simulink model "AFS_VDDrftComp"  (R2016b)
settings: configuration reference "CodeGenConfigSet" (kept outside this file)
values from neighbouring files (symbols this model uses):
  AFS_aOvrnAdjMax_C = Calibration.Parameter    [init_AFS_VDDrftComp.m]    (also in init_AFS_VDDrftComp_SIL.m = Simulink.Parameter)
  AFS_aOvrnAdjMin_C = Calibration.Parameter    [init_AFS_VDDrftComp.m]    (also in init_AFS_VDDrftComp_SIL.m = Simulink.Parameter)
  AFS_dmIdlAirMsLim_C = Calibration.Parameter    [init_AFS_VDDrftComp.m]    (also in init_AFS_VDDrftComp_SIL.m = Simulink.Parameter)
  AFS_dmLdAirMsLim_C = Calibration.Parameter    [init_AFS_VDDrftComp.m]    (also in init_AFS_VDDrftComp_SIL.m = Simulink.Parameter)
  AFS_dnEngLdAdjThresHi_C = Calibration.Parameter    [init_AFS_VDDrftComp.m]    (also in init_AFS_VDDrftComp_SIL.m = Simulink.Parameter)
  AFS_dpLdAdjThresHi_C = Calibration.Parameter    [init_AFS_VDDrftComp.m]    (also in init_AFS_VDDrftComp_SIL.m = Simulink.Parameter)
  AFS_dqLdAdjThresHi_C = Calibration.Parameter    [init_AFS_VDDrftComp.m]    (also in init_AFS_VDDrftComp_SIL.m = Simulink.Parameter)
  AFS_drWtPenDetThresHi_C = Calibration.Parameter    [init_AFS_VDDrftComp.m]    (also in init_AFS_VDDrftComp_SIL.m = Simulink.Parameter)
  AFS_facAdjPlausDiff_C = Calibration.Parameter    [init_AFS_VDDrftComp.m]    (also in init_AFS_VDDrftComp_SIL.m = Simulink.Parameter)
  AFS_facAirMsPT1_C = Calibration.Parameter    [init_AFS_VDDrftComp.m]    (also in init_AFS_VDDrftComp_SIL.m = Simulink.Parameter)
  AFS_facBstPresPT1_C = Calibration.Parameter    [init_AFS_VDDrftComp.m]    (also in init_AFS_VDDrftComp_SIL.m = Simulink.Parameter)
  AFS_facCorExtpIdl_CUR = Calibration.Parameter    [init_AFS_VDDrftComp.m]    (also in init_AFS_VDDrftComp_SIL.m = Simulink.Parameter)
  AFS_facCorExtpIdl_CURX = Calibration.Parameter    [init_AFS_VDDrftComp.m]    (also in init_AFS_VDDrftComp_SIL.m = Simulink.Parameter)
  AFS_facCorExtpLd_CUR = Calibration.Parameter    [init_AFS_VDDrftComp.m]    (also in init_AFS_VDDrftComp_SIL.m = Simulink.Parameter)
  AFS_facCorExtpLd_CURX = Calibration.Parameter    [init_AFS_VDDrftComp.m]    (also in init_AFS_VDDrftComp_SIL.m = Simulink.Parameter)
  AFS_facCorFacPT1_C = Calibration.Parameter    [init_AFS_VDDrftComp.m]    (also in init_AFS_VDDrftComp_SIL.m = Simulink.Parameter)
  AFS_facIdlAdjPlausMax_C = Calibration.Parameter    [init_AFS_VDDrftComp.m]    (also in init_AFS_VDDrftComp_SIL.m = Simulink.Parameter)
  AFS_facIdlAdjValMax_C = Calibration.Parameter    [init_AFS_VDDrftComp.m]    (also in init_AFS_VDDrftComp_SIL.m = Simulink.Parameter)
  AFS_facIdlAdjValMin_C = Calibration.Parameter    [init_AFS_VDDrftComp.m]    (also in init_AFS_VDDrftComp_SIL.m = Simulink.Parameter)
  AFS_facIdlAdjValStepLim_C = Calibration.Parameter    [init_AFS_VDDrftComp.m]    (also in init_AFS_VDDrftComp_SIL.m = Simulink.Parameter)
  AFS_facLdAdjPlausMin_C = Calibration.Parameter    [init_AFS_VDDrftComp.m]    (also in init_AFS_VDDrftComp_SIL.m = Simulink.Parameter)
  AFS_facLdAdjValMax_C = Calibration.Parameter    [init_AFS_VDDrftComp.m]    (also in init_AFS_VDDrftComp_SIL.m = Simulink.Parameter)
  AFS_facLdAdjValMin_C = Calibration.Parameter    [init_AFS_VDDrftComp.m]    (also in init_AFS_VDDrftComp_SIL.m = Simulink.Parameter)
  AFS_facLdAdjValStepLim_C = Calibration.Parameter    [init_AFS_VDDrftComp.m]    (also in init_AFS_VDDrftComp_SIL.m = Simulink.Parameter)
  AFS_facLoThresIdlAdjVal_C = Calibration.Parameter    [init_AFS_VDDrftComp.m]    (also in init_AFS_VDDrftComp_SIL.m = Simulink.Parameter)
  AFS_facLoThresLdAdjVal_C = Calibration.Parameter    [init_AFS_VDDrftComp.m]    (also in init_AFS_VDDrftComp_SIL.m = Simulink.Parameter)
  AFS_facnEngPT1_C = Calibration.Parameter    [init_AFS_VDDrftComp.m]    (also in init_AFS_VDDrftComp_SIL.m = Simulink.Parameter)
  AFS_facQntCurrPT1_C = Calibration.Parameter    [init_AFS_VDDrftComp.m]    (also in init_AFS_VDDrftComp_SIL.m = Simulink.Parameter)
  AFS_facWtPenDetPT1_C = Calibration.Parameter    [init_AFS_VDDrftComp.m]    (also in init_AFS_VDDrftComp_SIL.m = Simulink.Parameter)
  AFS_nAvrgIdlAdjThresHi_C = Calibration.Parameter    [init_AFS_VDDrftComp.m]    (also in init_AFS_VDDrftComp_SIL.m = Simulink.Parameter)
  AFS_nAvrgIdlAdjThresLo_C = Calibration.Parameter    [init_AFS_VDDrftComp.m]    (also in init_AFS_VDDrftComp_SIL.m = Simulink.Parameter)
  AFS_nOvrnAdjMax_C = Calibration.Parameter    [init_AFS_VDDrftComp.m]    (also in init_AFS_VDDrftComp_SIL.m = Simulink.Parameter)
  AFS_nOvrnAdjMin_C = Calibration.Parameter    [init_AFS_VDDrftComp.m]    (also in init_AFS_VDDrftComp_SIL.m = Simulink.Parameter)
  AFS_numAirDrftComp_C = Calibration.Parameter    [init_AFS_VDDrftComp.m]    (also in init_AFS_VDDrftComp_SIL.m = Simulink.Parameter)
  AFS_numEnvTemp_C = Calibration.Parameter    [init_AFS_VDDrftComp.m]    (also in init_AFS_VDDrftComp_SIL.m = Simulink.Parameter)
  AFS_numOvrnAdjGearMin_C = Calibration.Parameter    [init_AFS_VDDrftComp.m]    (also in init_AFS_VDDrftComp_SIL.m = Simulink.Parameter)
  AFS_pBstAtmDiffLim_C = Calibration.Parameter    [init_AFS_VDDrftComp.m]    (also in init_AFS_VDDrftComp_SIL.m = Simulink.Parameter)
  AFS_pBstLdAdjThresHi_C = Calibration.Parameter    [init_AFS_VDDrftComp.m]    (also in init_AFS_VDDrftComp_SIL.m = Simulink.Parameter)
  AFS_pBstLdAdjThresLo_C = Calibration.Parameter    [init_AFS_VDDrftComp.m]    (also in init_AFS_VDDrftComp_SIL.m = Simulink.Parameter)
  AFS_qCurrIdlAdjThresHi_C = Calibration.Parameter    [init_AFS_VDDrftComp.m]    (also in init_AFS_VDDrftComp_SIL.m = Simulink.Parameter)
  AFS_qCurrIdlAdjThresLo_C = Calibration.Parameter    [init_AFS_VDDrftComp.m]    (also in init_AFS_VDDrftComp_SIL.m = Simulink.Parameter)
  AFS_qWinLdAdjThresHi_CUR = Calibration.Parameter    [init_AFS_VDDrftComp.m]    (also in init_AFS_VDDrftComp_SIL.m = Simulink.Parameter)
  AFS_qWinLdAdjThresHi_CURX = Calibration.Parameter    [init_AFS_VDDrftComp.m]    (also in init_AFS_VDDrftComp_SIL.m = Simulink.Parameter)
  AFS_qWinLdAdjThresLo_CUR = Calibration.Parameter    [init_AFS_VDDrftComp.m]    (also in init_AFS_VDDrftComp_SIL.m = Simulink.Parameter)
  AFS_qWinLdAdjThresLo_CURX = Calibration.Parameter    [init_AFS_VDDrftComp.m]    (also in init_AFS_VDDrftComp_SIL.m = Simulink.Parameter)
  AFS_swtAdjPlausLim_C = Calibration.Parameter    [init_AFS_VDDrftComp.m]    (also in init_AFS_VDDrftComp_SIL.m = Simulink.Parameter)
  AFS_swtAirMsCorRls_C = Calibration.Parameter    [init_AFS_VDDrftComp.m]    (also in init_AFS_VDDrftComp_SIL.m = Simulink.Parameter)
  AFS_swtLdAdjSel_C = Calibration.Parameter    [init_AFS_VDDrftComp.m]    (also in init_AFS_VDDrftComp_SIL.m = Simulink.Parameter)
  AFS_tAirAdjRlsThresHi_C = Calibration.Parameter    [init_AFS_VDDrftComp.m]    (also in init_AFS_VDDrftComp_SIL.m = Simulink.Parameter)
  AFS_tAirAdjRlsThresLo_C = Calibration.Parameter    [init_AFS_VDDrftComp.m]    (also in init_AFS_VDDrftComp_SIL.m = Simulink.Parameter)
  AFS_tEnvAdjRlsThresHi_C = Calibration.Parameter    [init_AFS_VDDrftComp.m]    (also in init_AFS_VDDrftComp_SIL.m = Simulink.Parameter)
  AFS_tEnvAdjRlsThresLo_C = Calibration.Parameter    [init_AFS_VDDrftComp.m]    (also in init_AFS_VDDrftComp_SIL.m = Simulink.Parameter)
  AFS_tiAdjRlsDel_C = Calibration.Parameter    [init_AFS_VDDrftComp.m]    (also in init_AFS_VDDrftComp_SIL.m = Simulink.Parameter)
  AFS_tiIdlAdjRlsDeb = Calibration.Parameter    [init_AFS_VDDrftComp.m]    (also in init_AFS_VDDrftComp_SIL.m = Simulink.Parameter)
  AFS_tiLdAdjRlsDeb = Calibration.Parameter    [init_AFS_VDDrftComp.m]    (also in init_AFS_VDDrftComp_SIL.m = Simulink.Parameter)
  AFS_tiStrtDelAdjRls_C = Calibration.Parameter    [init_AFS_VDDrftComp.m]    (also in init_AFS_VDDrftComp_SIL.m = Simulink.Parameter)
  AFS_tiWtPenDeb = Calibration.Parameter    [init_AFS_VDDrftComp.m]    (also in init_AFS_VDDrftComp_SIL.m = Simulink.Parameter)
  AFS_vOvrnAdjMin_C = Calibration.Parameter    [init_AFS_VDDrftComp.m]    (also in init_AFS_VDDrftComp_SIL.m = Simulink.Parameter)
  AFS_vVehLdAdjThresHi_C = Calibration.Parameter    [init_AFS_VDDrftComp.m]    (also in init_AFS_VDDrftComp_SIL.m = Simulink.Parameter)
  AFS_vVehLdAdjThresLo_C = Calibration.Parameter    [init_AFS_VDDrftComp.m]    (also in init_AFS_VDDrftComp_SIL.m = Simulink.Parameter)
  AIRCTL_DRFTCOMP = fi(5,State_uint8)    [init_AFS_VDDrftComp.m]    (also in init_AFS_VDDrftComp_SIL.m)
undefined symbols (not defined in the file or in its folder): AFS_VDDrftComp_DT, Switch_conv
libraries: simulink x82, CXLib x13
(part 2 of 2)

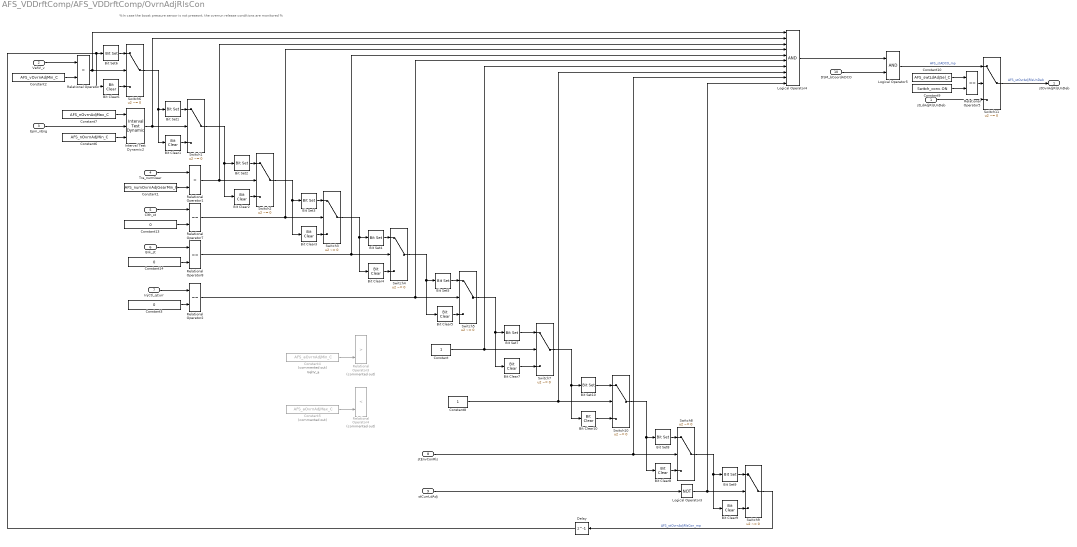
== system AFS_VDDrftComp/AFS_VDDrftComp/OvrnAdjRlsCon ==
  note: VehV_a
  note: %In case the boost pressure sensor is not presesnt, the overrun release conditions are monitored %
  stLdAdjRlsUnDeb : Inport
  VehV_v : Inport  Port=2
  Epm_nEng : Inport  Port=3
  Tra_numGear : Inport  Port=4
  Clth_st : Inport  Port=5
  Brk_st : Inport  Port=6
  InjCtl_qCurr : Inport  Port=7
  stEnvConRls : Inport  Port=8
  stCurrLdAdj : Inport  Port=9
  DSM_bCoordADCO : Inport  Port=10
  Bit Clear1 : simulink/Logic and Bit Operations/Bit Clear  iBit=1
  Bit Clear10 : simulink/Logic and Bit Operations/Bit Clear  iBit=7
  Bit Clear2 : simulink/Logic and Bit Operations/Bit Clear  iBit=2
  Bit Clear3 : simulink/Logic and Bit Operations/Bit Clear  iBit=3
  Bit Clear4 : simulink/Logic and Bit Operations/Bit Clear  iBit=4
  Bit Clear5 : simulink/Logic and Bit Operations/Bit Clear  iBit=5
  Bit Clear6 : simulink/Logic and Bit Operations/Bit Clear  iBit=0
  Bit Clear7 : simulink/Logic and Bit Operations/Bit Clear  iBit=6
  Bit Clear8 : simulink/Logic and Bit Operations/Bit Clear  iBit=8
  Bit Clear9 : simulink/Logic and Bit Operations/Bit Clear  iBit=9
  Bit Set1 : simulink/Logic and Bit Operations/Bit Set  iBit=1
  Bit Set10 : simulink/Logic and Bit Operations/Bit Set  iBit=7
  Bit Set2 : simulink/Logic and Bit Operations/Bit Set  iBit=2
  Bit Set3 : simulink/Logic and Bit Operations/Bit Set  iBit=3
  Bit Set4 : simulink/Logic and Bit Operations/Bit Set  iBit=4
  Bit Set5 : simulink/Logic and Bit Operations/Bit Set  iBit=5
  Bit Set6 : simulink/Logic and Bit Operations/Bit Set  iBit=0
  Bit Set7 : simulink/Logic and Bit Operations/Bit Set  iBit=6
  Bit Set8 : simulink/Logic and Bit Operations/Bit Set  iBit=8
  Bit Set9 : simulink/Logic and Bit Operations/Bit Set  iBit=9
  Constant : Constant  OutDataTypeStr=boolean
  Constant1 : Constant  Value=AFS_numOvrnAdjGearMin_C
  Constant10 : Constant  Value=AFS_swtLdAdjSel_C
  Constant13 : Constant  Value=0  OutDataTypeStr=Inherit: Inherit via back propagation
  Constant14 : Constant  Value=0  OutDataTypeStr=Inherit: Inherit via back propagation
  Constant2 : Constant  Value=AFS_vOvrnAdjMin_C
  Constant3 : Constant  Value=0  OutDataTypeStr=Inherit: Inherit via back propagation
  Constant4 : Constant  Commented=on  Value=AFS_aOvrnAdjMin_C
  Constant5 : Constant  Commented=on  Value=AFS_aOvrnAdjMax_C
  Constant6 : Constant  Value=AFS_nOvrnAdjMin_C
  Constant7 : Constant  Value=AFS_nOvrnAdjMax_C
  Constant8 : Constant  OutDataTypeStr=boolean
  Constant9 : Constant  Value=Switch_conv.ON
  Delay : Delay  DelayLength=1  InitialCondition=0
  Interval Test Dynamic2 : simulink/Logic and Bit Operations/Interval Test Dynamic  IntervalClosedRight=off  IntervalClosedLeft=off  OutDataTypeStr=boolean
  Logical Operator3 : Logic  Operator=NOT  Inputs=5  AllPortsSameDT=off  OutDataTypeStr=boolean
  Logical Operator4 : Logic  Inputs=10  AllPortsSameDT=off  OutDataTypeStr=boolean
  Logical Operator5 : Logic  AllPortsSameDT=off  OutDataTypeStr=boolean
  Relational Operator : RelationalOperator  Operator=>  OutDataTypeStr=boolean  RndMeth=Simplest
  Relational Operator1 : RelationalOperator  Operator=>  OutDataTypeStr=boolean  RndMeth=Simplest
  Relational Operator2 : RelationalOperator  Operator===  OutDataTypeStr=boolean  RndMeth=Simplest  InputSameDT=on
  Relational Operator3 : RelationalOperator  Commented=on  Operator=>  OutDataTypeStr=boolean  RndMeth=Simplest  InputSameDT=on
  Relational Operator4 : RelationalOperator  Commented=on  Operator=<  OutDataTypeStr=boolean  RndMeth=Simplest  InputSameDT=on
  Relational Operator5 : RelationalOperator  Operator===  OutDataTypeStr=boolean  RndMeth=Simplest
  Relational Operator7 : RelationalOperator  Operator===  OutDataTypeStr=boolean  RndMeth=Simplest  InputSameDT=on
  Relational Operator8 : RelationalOperator  Operator===  OutDataTypeStr=boolean  RndMeth=Simplest  InputSameDT=on
  Switch{1..11} (11 alike) : Switch  Criteria=u2 ~= 0  OutDataTypeStr=Inherit: Inherit via back propagation  SaturateOnIntegerOverflow=on
  stOvrAdjRlsUnDeb : Outport
  wires:
  Constant14/1 -> Relational Operator8/2
  Brk_st/1 -> Relational Operator8/1
  Constant13/1 -> Relational Operator7/2
  Switch11/1 -> stOvrAdjRlsUnDeb/1  "AFS_stOvrAdjRlsUnDeb"
  Constant10/1 -> Relational Operator5/1
  Relational Operator5/1 -> Switch11/2
  Constant9/1 -> Relational Operator5/2
  stLdAdjRlsUnDeb/1 -> Switch11/3
  Logical Operator5/1 -> Switch11/1  "AFS_stADCO_mp"
  Logical Operator4/1 -> Logical Operator5/1
  Delay/1 -> Bit Set6/1, Bit Clear6/1
  Switch9/1 -> Delay/1  "AFS_stOvrnAdjRlsCon_mp"
  Switch10/1 -> Bit Set8/1, Bit Clear8/1
  Constant5/1 -> Relational Operator4/2
  Switch7/1 -> Bit Clear10/1, Bit Set10/1
  Bit Set10/1 -> Switch10/1
  Bit Clear10/1 -> Switch10/3
  Switch8/1 -> Bit Clear9/1, Bit Set9/1
  Logical Operator3/1 -> Switch9/2, Logical Operator4/10
  Bit Set9/1 -> Switch9/1
  Bit Clear9/1 -> Switch9/3
  stCurrLdAdj/1 -> Logical Operator3/1
  stEnvConRls/1 -> Switch8/2, Logical Operator4/9
  Bit Set8/1 -> Switch8/1
  Bit Clear8/1 -> Switch8/3
  Switch5/1 -> Bit Set7/1, Bit Clear7/1
  Bit Set7/1 -> Switch7/1
  Bit Clear7/1 -> Switch7/3
  Constant4/1 -> Relational Operator3/2
  Switch4/1 -> Bit Clear5/1, Bit Set5/1
  Relational Operator2/1 -> Switch5/2, Logical Operator4/6
  Bit Set5/1 -> Switch5/1
  Bit Clear5/1 -> Switch5/3
  InjCtl_qCurr/1 -> Relational Operator2/1
  Constant3/1 -> Relational Operator2/2
  Switch3/1 -> Bit Set4/1, Bit Clear4/1
  Relational Operator8/1 -> Switch4/2, Logical Operator4/5
  Bit Set4/1 -> Switch4/1
  Bit Clear4/1 -> Switch4/3
  Switch2/1 -> Bit Clear3/1, Bit Set3/1
  Relational Operator7/1 -> Switch3/2, Logical Operator4/4
  Bit Set3/1 -> Switch3/1
  Bit Clear3/1 -> Switch3/3
  Clth_st/1 -> Relational Operator7/1
  Switch1/1 -> Bit Set2/1, Bit Clear2/1
  Relational Operator1/1 -> Switch2/2, Logical Operator4/3
  Bit Set2/1 -> Switch2/1
  Bit Clear2/1 -> Switch2/3
  Tra_numGear/1 -> Relational Operator1/1
  Constant1/1 -> Relational Operator1/2
  Switch6/1 -> Bit Set1/1, Bit Clear1/1
  Interval Test Dynamic2/1 -> Switch1/2, Logical Operator4/2
  Bit Set1/1 -> Switch1/1
  Bit Clear1/1 -> Switch1/3
  Epm_nEng/1 -> Interval Test Dynamic2/2
  Constant6/1 -> Interval Test Dynamic2/3
  Constant7/1 -> Interval Test Dynamic2/1
  Relational Operator/1 -> Switch6/2, Logical Operator4/1
  Bit Set6/1 -> Switch6/1
  Bit Clear6/1 -> Switch6/3
  VehV_v/1 -> Relational Operator/1
  Constant2/1 -> Relational Operator/2
  DSM_bCoordADCO/1 -> Logical Operator5/2
  Constant/1 -> Logical Operator4/7, Switch7/2
  Constant8/1 -> Logical Operator4/8, Switch10/2

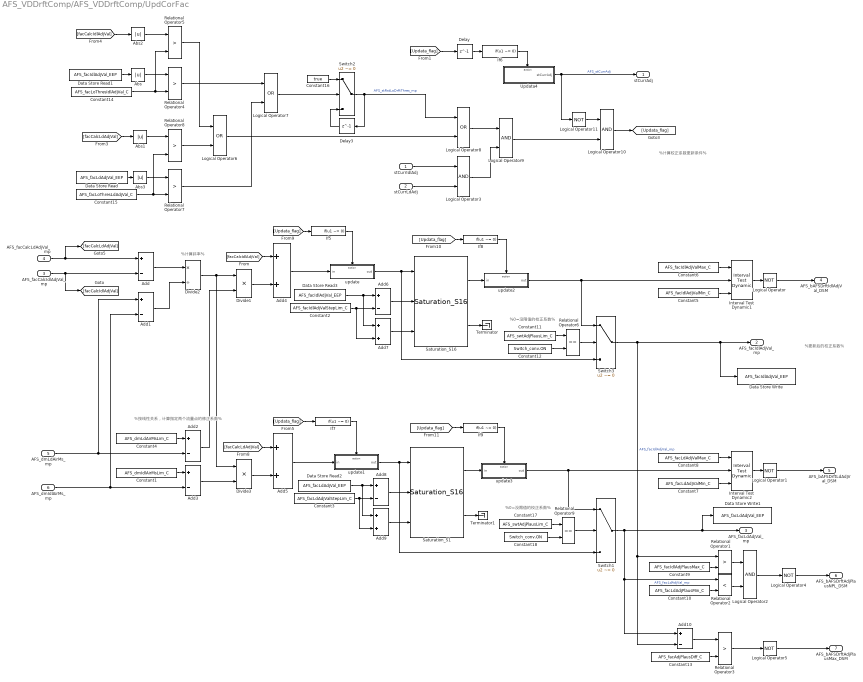
== system AFS_VDDrftComp/AFS_VDDrftComp/UpdCorFac ==
  note: %0=没限值的校正系数%
  note: %计算斜率%
  note: %0=没限值的校正系数%
  note: %计算校正系数更新条件%
  note: %更新后的校正系数%
  note: %按线性关系，计算指定两个流量点的修正系数%
  stCurrIdlAdj : Inport
  stCurrLdAdj : Inport  Port=2
  AFS_facCalcIdlAdjVal_mp : Inport  Port=3
  AFS_facCalcLdAdjVal_mp : Inport  Port=4
  AFS_dmLdAirMs_mp : Inport  Port=5
  AFS_dmIdlAirMs_mp : Inport  Port=6
  Abs{,1..3} (4 alike) : Abs  SaturateOnIntegerOverflow=on
  Add{,2..3,6,8,10} (6 alike) : Sum  Inputs=+-  OutDataTypeStr=Inherit: Inherit via back propagation  SaturateOnIntegerOverflow=on  InputSameDT=on
  Add1 : Sum  Inputs=+-  SaturateOnIntegerOverflow=on  InputSameDT=on
  Add{4..5,7,9} (4 alike) : Sum  OutDataTypeStr=Inherit: Inherit via back propagation  SaturateOnIntegerOverflow=on  InputSameDT=on
  Constant1 : Constant  Value=AFS_dmIdlAirMsLim_C
  Constant10 : Constant  Value=AFS_facLdAdjPlausMin_C
  Constant11 : Constant  Value=AFS_swtAdjPlausLim_C
  Constant12 : Constant  Value=Switch_conv.ON
  Constant13 : Constant  Value=AFS_facAdjPlausDiff_C
  Constant14 : Constant  Value=AFS_facLoThresIdlAdjVal_C
  Constant15 : Constant  Value=AFS_facLoThresLdAdjVal_C
  Constant16 : Constant  Value=true  OutDataTypeStr=Inherit: Inherit via back propagation
  Constant17 : Constant  Value=AFS_swtAdjPlausLim_C
  Constant18 : Constant  Value=Switch_conv.ON
  Constant2 : Constant  Value=AFS_facIdlAdjValStepLim_C
  Constant3 : Constant  Value=AFS_facLdAdjValStepLim_C
  Constant4 : Constant  Value=AFS_dmLdAirMsLim_C
  Constant5 : Constant  Value=AFS_facIdlAdjValMin_C
  Constant6 : Constant  Value=AFS_facIdlAdjValMax_C
  Constant7 : Constant  Value=AFS_facLdAdjValMin_C
  Constant8 : Constant  Value=AFS_facLdAdjValMax_C
  Constant9 : Constant  Value=AFS_facIdlAdjPlausMax_C
  Data Store Read : DataStoreRead  DataStoreName=AFS_facLdAdjVal_EEP
  Data Store Read1 : DataStoreRead  DataStoreName=AFS_facIdlAdjVal_EEP
  Data Store Read2 : DataStoreRead  DataStoreName=AFS_facLdAdjVal_EEP
  Data Store Read3 : DataStoreRead  DataStoreName=AFS_facIdlAdjVal_EEP
  Data Store Write : DataStoreWrite  DataStoreName=AFS_facIdlAdjVal_EEP
  Data Store Write1 : DataStoreWrite  DataStoreName=AFS_facLdAdjVal_EEP
  Delay : Delay  DelayLength=1  InitialCondition=0
  Delay3 : Delay  DelayLength=1  InitialCondition=0
  Divide1 : Product  Inputs=**  OutDataTypeStr=Inherit: Inherit via back propagation  SaturateOnIntegerOverflow=on
  Divide2 : Product  Inputs=*/  SaturateOnIntegerOverflow=on
  Divide3 : Product  Inputs=**  OutDataTypeStr=Inherit: Inherit via back propagation  SaturateOnIntegerOverflow=on
  If{5..9} (5 alike) : If  IfExpression=u1 ~= 0  ShowElse=off
  Interval Test Dynamic1 : simulink/Logic and Bit Operations/Interval Test Dynamic  IntervalClosedRight=on  IntervalClosedLeft=on  OutDataTypeStr=boolean
  Interval Test Dynamic2 : simulink/Logic and Bit Operations/Interval Test Dynamic  IntervalClosedRight=on  IntervalClosedLeft=on  OutDataTypeStr=boolean
  Logical Operator{,1,4..5,11} (5 alike) : Logic  Operator=NOT  AllPortsSameDT=off  OutDataTypeStr=boolean
  Logical Operator{2..3,9..10} (4 alike) : Logic  OutDataTypeStr=boolean
  Logical Operator6 : Logic  Operator=OR  OutDataTypeStr=boolean
  Logical Operator7 : Logic  Operator=OR  OutDataTypeStr=boolean
  Logical Operator8 : Logic  Operator=OR  OutDataTypeStr=boolean
  Relational Operator{1,3..5,7..8} (6 alike) : RelationalOperator  Operator=>  OutDataTypeStr=boolean  RndMeth=Simplest  InputSameDT=on
  Relational Operator2 : RelationalOperator  Operator=<  OutDataTypeStr=boolean  RndMeth=Simplest  InputSameDT=on
  Relational Operator6 : RelationalOperator  Operator===  OutDataTypeStr=boolean  RndMeth=Simplest  InputSameDT=on
  Relational Operator9 : RelationalOperator  Operator===  OutDataTypeStr=boolean  RndMeth=Simplest  InputSameDT=on
  Saturation_S1 : CXLib/Saturation_S16
  Saturation_S16 : CXLib/Saturation_S16
  Switch1 : Switch  Criteria=u2 ~= 0  OutDataTypeStr=Inherit: Inherit via back propagation  SaturateOnIntegerOverflow=on  InputSameDT=on
  Switch2 : Switch  Criteria=u2 ~= 0  OutDataTypeStr=Inherit: Inherit via back propagation  SaturateOnIntegerOverflow=on  InputSameDT=on
  Switch3 : Switch  Criteria=u2 ~= 0  OutDataTypeStr=Inherit: Inherit via back propagation  SaturateOnIntegerOverflow=on  InputSameDT=on
  Terminator : Terminator
  Terminator1 : Terminator
  Updata4 : Subsystem  TreatAsAtomicUnit=on
  update : Subsystem  TreatAsAtomicUnit=on
  update1 : Subsystem  TreatAsAtomicUnit=on
  update2 : Subsystem  TreatAsAtomicUnit=on
  update3 : Subsystem  TreatAsAtomicUnit=on
  stCurrAdj : Outport
  AFS_facIdlAdjVal_mp : Outport  Port=2
  AFS_facLdAdjVal_mp : Outport  Port=3
  AFS_bAFSDrftIdlAdjVal_DSM : Outport  Port=4
  AFS_bAFSDrftLdAdjVal_DSM : Outport  Port=5
  AFS_bAFSDrftAdjPlausNPL_DSM : Outport  Port=6
  AFS_bAFSDrftAdjPlausMax_DSM : Outport  Port=7
  wires:
  Delay/1 -> If6/1
  Logical Operator11/1 -> Logical Operator10/1
  [Updata_flag] -> Delay/1
  Relational Operator9/1 -> Switch1/2
  Constant17/1 -> Relational Operator9/1
  Constant18/1 -> Relational Operator9/2
  Saturation_S1/1 -> update3/1(in)
  If9/1 -> update3/Action
  Saturation_S16/1 -> update2/1(in)
  If8/1 -> update2/Action
  [Updata_flag] -> If9/1
  [Updata_flag] -> If8/1
  Add9/1 -> Saturation_S1/3
  Add8/1 -> Saturation_S1/2
  update1/1(out) -> Saturation_S1/1, Switch1/3
  Add5/1 -> update1/1(in)
  [Updata_flag] -> If7/1
  If7/1 -> update1/Action
  [facCalcIdlAdjVal] -> Add4/1
  [facCalcLdAdjVal] -> Add5/1
  [Updata_flag] -> If5/1
  If5/1 -> update/Action
  Delay3/1 -> Switch2/3
  Constant16/1 -> Switch2/1
  [facCalcIdlAdjVal] -> Abs2/1
  [facCalcLdAdjVal] -> Abs1/1
  Updata4/1(stCurrAdj) -> stCurrAdj/1, Logical Operator11/1  "AFS_stCurrAdj"
  If6/1 -> Updata4/Action
  Logical Operator10/1 -> [Updata_flag]
  Logical Operator9/1 -> Logical Operator10/2
  Logical Operator3/1 -> Logical Operator9/2
  Logical Operator8/1 -> Logical Operator9/1
  Logical Operator6/1 -> Logical Operator8/2
  Switch2/1 -> Logical Operator8/1, Delay3/1  "AFS_stRstLoDrftThres_mp"
  Logical Operator7/1 -> Switch2/2
  Relational Operator7/1 -> Logical Operator7/2
  Relational Operator4/1 -> Logical Operator7/1
  Relational Operator5/1 -> Logical Operator6/1
  Relational Operator8/1 -> Logical Operator6/2
  Abs3/1 -> Relational Operator7/1
  Abs2/1 -> Relational Operator5/1
  Abs1/1 -> Relational Operator8/1
  Data Store Read/1 -> Abs3/1
  Constant15/1 -> Relational Operator7/2, Relational Operator8/2
  Constant14/1 -> Relational Operator4/2, Relational Operator5/2
  Abs/1 -> Relational Operator4/1
  Data Store Read1/1 -> Abs/1
  Logical Operator5/1 -> AFS_bAFSDrftAdjPlausMax_DSM/1
  Relational Operator3/1 -> Logical Operator5/1
  Constant13/1 -> Relational Operator3/2
  Add10/1 -> Relational Operator3/1
  Logical Operator2/1 -> Logical Operator4/1
  Relational Operator2/1 -> Logical Operator2/2
  Relational Operator1/1 -> Logical Operator2/1
  Constant10/1 -> Relational Operator2/2
  Switch1/1 -> Relational Operator2/1, Add10/1, Data Store Write1/1, AFS_facLdAdjVal_mp/1  "AFS_facLdAdjVal_mp"
  Constant9/1 -> Relational Operator1/2
  Switch3/1 -> Relational Operator1/1, Add10/2, Data Store Write/1, AFS_facIdlAdjVal_mp/1  "AFS_facIdlAdjVal_mp"
  Interval Test Dynamic2/1 -> Logical Operator1/1
  Constant7/1 -> Interval Test Dynamic2/3
  Constant8/1 -> Interval Test Dynamic2/1
  Logical Operator/1 -> AFS_bAFSDrftIdlAdjVal_DSM/1
  Interval Test Dynamic1/1 -> Logical Operator/1
  Constant5/1 -> Interval Test Dynamic1/3
  Constant6/1 -> Interval Test Dynamic1/1
  update/1(out) -> Saturation_S16/1, Switch3/3
  update3/1(out) -> Interval Test Dynamic2/2, Switch1/1
  update2/1(out) -> Switch3/1, Interval Test Dynamic1/2
  Relational Operator6/1 -> Switch3/2
  Constant11/1 -> Relational Operator6/1
  Constant12/1 -> Relational Operator6/2
  Saturation_S1/2 -> Terminator1/1
  Saturation_S16/2 -> Terminator/1
  Constant3/1 -> Add8/2, Add9/2
  Data Store Read2/1 -> Add8/1, Add9/1
  Add7/1 -> Saturation_S16/3
  Add6/1 -> Saturation_S16/2
  Constant2/1 -> Add7/2, Add6/2
  Data Store Read3/1 -> Add6/1, Add7/1
  Add4/1 -> update/1(in)
  Divide3/1 -> Add5/2
  Add3/1 -> Divide3/2
  Divide1/1 -> Add4/2
  Add2/1 -> Divide1/2
  Divide2/1 -> Divide3/1, Divide1/1
  Constant1/1 -> Add3/1
  Constant4/1 -> Add2/1
  Add1/1 -> Divide2/2
  Add/1 -> Divide2/1
  AFS_dmIdlAirMs_mp/1 -> Add3/2, Add1/2
  AFS_dmLdAirMs_mp/1 -> Add1/1, Add2/2
  AFS_facCalcIdlAdjVal_mp/1 -> [facCalcIdlAdjVal], Add/2
  AFS_facCalcLdAdjVal_mp/1 -> Add/1, [facCalcLdAdjVal]
  stCurrLdAdj/1 -> Logical Operator3/2
  stCurrIdlAdj/1 -> Logical Operator3/1
  Logical Operator1/1 -> AFS_bAFSDrftLdAdjVal_DSM/1
  Logical Operator4/1 -> AFS_bAFSDrftAdjPlausNPL_DSM/1

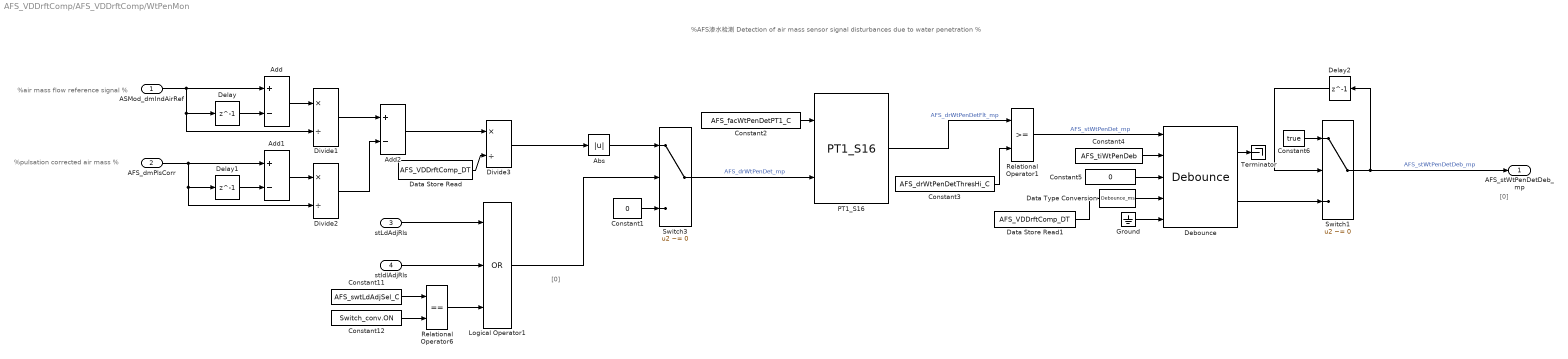
== system AFS_VDDrftComp/AFS_VDDrftComp/WtPenMon ==
  note: %AFS渗水检测
      | Detection of air mass sensor signal disturbances due to water penetration %
  note: %pulsation corrected air mass %
  note: %air mass flow reference signal %
  note: [0]
  note: [0]
  ASMod_dmIndAirRef : Inport
  AFS_dmPlsCorr : Inport  Port=2
  stLdAdjRls : Inport  Port=3
  stIdlAdjRls : Inport  Port=4
  Abs : Abs  SaturateOnIntegerOverflow=on
  Add : Sum  Inputs=+-  OutDataTypeStr=Inherit: Inherit via back propagation  SaturateOnIntegerOverflow=on  InputSameDT=on
  Add1 : Sum  Inputs=+-  OutDataTypeStr=Inherit: Inherit via back propagation  SaturateOnIntegerOverflow=on  InputSameDT=on
  Add2 : Sum  Inputs=+-  SaturateOnIntegerOverflow=on  InputSameDT=on
  Constant1 : Constant  Value=0  OutDataTypeStr=Rmp_1_s
  Constant11 : Constant  Value=AFS_swtLdAdjSel_C
  Constant12 : Constant  Value=Switch_conv.ON
  Constant2 : Constant  Value=AFS_facWtPenDetPT1_C
  Constant3 : Constant  Value=AFS_drWtPenDetThresHi_C
  Constant4 : Constant  Value=AFS_tiWtPenDeb
  Constant5 : Constant  Value=0  OutDataTypeStr=Debounce_ms
  Constant6 : Constant  Value=true  OutDataTypeStr=Inherit: Inherit via back propagation
  Data Store Read : DataStoreRead  DataStoreName=AFS_VDDrftComp_DT
  Data Store Read1 : DataStoreRead  DataStoreName=AFS_VDDrftComp_DT
  Data Type Conversion : DataTypeConversion  OutDataTypeStr=Debounce_ms
  Debounce : CXLib/Debounce
  Delay : Delay  DelayLength=1  InitialCondition=0
  Delay1 : Delay  DelayLength=1  InitialCondition=0
  Delay2 : Delay  DelayLength=1  InitialCondition=0
  Divide1 : Product  Inputs=*/  OutDataTypeStr=Factor  SaturateOnIntegerOverflow=on
  Divide2 : Product  Inputs=*/  OutDataTypeStr=Factor  SaturateOnIntegerOverflow=on
  Divide3 : Product  Inputs=*/  OutDataTypeStr=Inherit: Inherit via back propagation  SaturateOnIntegerOverflow=on
  Ground : Ground
  Logical Operator1 : Logic  Operator=OR  Inputs=3  OutDataTypeStr=boolean
  PT1_S16 : CXLib/PT1_S16
  Relational Operator1 : RelationalOperator  OutDataTypeStr=boolean  RndMeth=Simplest  InputSameDT=on
  Relational Operator6 : RelationalOperator  Operator===  OutDataTypeStr=boolean  RndMeth=Simplest
  Switch1 : Switch  Criteria=u2 ~= 0  OutDataTypeStr=Inherit: Inherit via back propagation  SaturateOnIntegerOverflow=on  InputSameDT=on
  Switch3 : Switch  Criteria=u2 ~= 0  OutDataTypeStr=Inherit: Inherit via back propagation  SaturateOnIntegerOverflow=on  InputSameDT=on
  Terminator : Terminator
  AFS_stWtPenDetDeb_mp : Outport
  wires:
  Debounce/1 -> Terminator/1
  Delay2/1 -> Switch1/2
  Switch1/1 -> Delay2/1, AFS_stWtPenDetDeb_mp/1  "AFS_stWtPenDetDeb_mp"
  Constant6/1 -> Switch1/1
  Debounce/2 -> Switch1/3
  Constant5/1 -> Debounce/3
  Constant4/1 -> Debounce/2
  Data Store Read1/1 -> Data Type Conversion/1
  Ground/1 -> Debounce/5
  Relational Operator1/1 -> Debounce/1  "AFS_stWtPenDet_mp"
  Constant2/1 -> PT1_S16/1
  Switch3/1 -> PT1_S16/2  "AFS_drWtPenDet_mp"
  Constant1/1 -> Switch3/3
  Logical Operator1/1 -> Switch3/2
  Relational Operator6/1 -> Logical Operator1/3
  Constant11/1 -> Relational Operator6/1
  Constant12/1 -> Relational Operator6/2
  Abs/1 -> Switch3/1
  Divide3/1 -> Abs/1
  Data Store Read/1 -> Divide3/2
  Add2/1 -> Divide3/1
  Divide2/1 -> Add2/2
  Add1/1 -> Divide2/1
  AFS_dmPlsCorr/1 -> Add1/1, Delay1/1, Divide2/2
  Delay1/1 -> Add1/2
  Divide1/1 -> Add2/1
  ASMod_dmIndAirRef/1 -> Add/1, Delay/1, Divide1/2
  Add/1 -> Divide1/1
  Delay/1 -> Add/2
  stIdlAdjRls/1 -> Logical Operator1/2
  stLdAdjRls/1 -> Logical Operator1/1
  PT1_S16/1 -> Relational Operator1/1  "AFS_drWtPenDetFlt_mp"
  Constant3/1 -> Relational Operator1/2
  Data Type Conversion/1 -> Debounce/4

== system AFS_VDDrftComp/AFS_VDDrftComp/ AdjRlsEnvCon/AFS_tAirDrftComp_mp ==
  TempSwt : Inport
  Air_tAFS_mp : Inport  Tag=deg  Description=Induction air temperature at the HFM  Port=2
  EnvT_t : Inport  Tag=deg  Description=Environmental temperature  Port=3
  Air_tIntkVUs : Inport  Tag=deg  Description=Intake air temperature upstream of the inlet valve  Port=4
  Data Type Conversion : DataTypeConversion  OutDataTypeStr=uint8
  Multiport Switch : MultiPortSwitch  DataPortOrder=Zero-based contiguous
  AFS_tAirDrftComp_mp : Outport  Tag=deg  Description=Engine temperature field
  wires:
  Multiport Switch/1 -> AFS_tAirDrftComp_mp/1
  Data Type Conversion/1 -> Multiport Switch/1
  TempSwt/1 -> Data Type Conversion/1
  Air_tIntkVUs/1 -> Multiport Switch/4
  Air_tAFS_mp/1 -> Multiport Switch/2
  EnvT_t/1 -> Multiport Switch/3

== system AFS_VDDrftComp/AFS_VDDrftComp/ AdjRlsEnvCon/AFS_tEnvTemp_mp ==
  TempSwt : Inport
  Air_tAFS_mp : Inport  Tag=deg  Description=Induction air temperature at the HFM  Port=2
  EnvT_t : Inport  Tag=deg  Description=Environmental temperature  Port=3
  Air_tIntkVUs : Inport  Tag=deg  Description=Intake air temperature upstream of the inlet valve  Port=4
  Data Type Conversion : DataTypeConversion  OutDataTypeStr=uint8
  Multiport Switch : MultiPortSwitch  DataPortOrder=Zero-based contiguous
  AFS_tEnvTemp_mp : Outport  Tag=deg  Description=Engine temperature field
  wires:
  Multiport Switch/1 -> AFS_tEnvTemp_mp/1
  Data Type Conversion/1 -> Multiport Switch/1
  TempSwt/1 -> Data Type Conversion/1
  Air_tIntkVUs/1 -> Multiport Switch/4
  Air_tAFS_mp/1 -> Multiport Switch/2
  EnvT_t/1 -> Multiport Switch/3

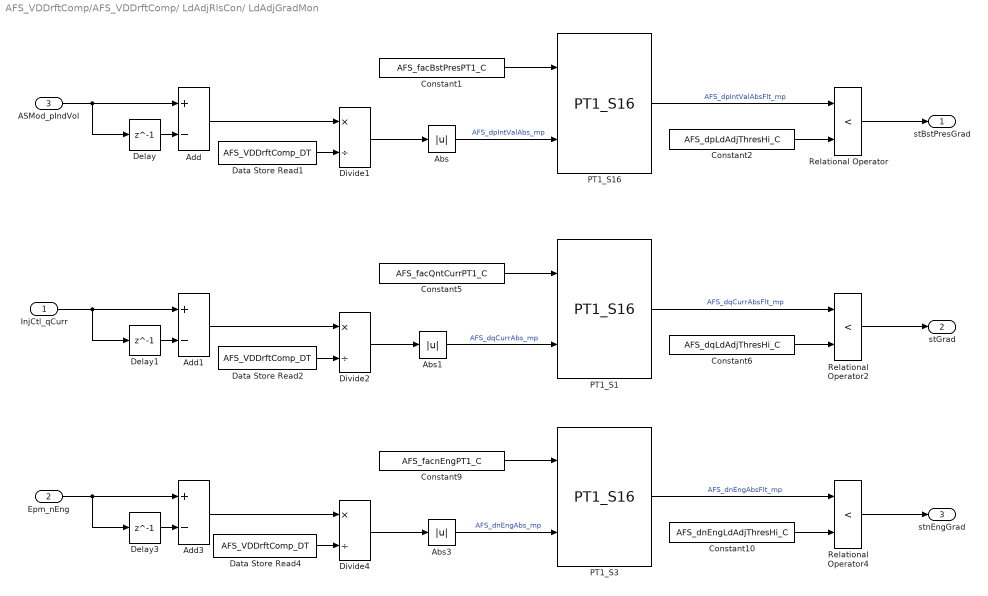
== system AFS_VDDrftComp/AFS_VDDrftComp/ LdAdjRlsCon/ LdAdjGradMon ==
  InjCtl_qCurr : Inport
  Epm_nEng : Inport  Port=2
  ASMod_pIndVol : Inport  Port=3
  Abs : Abs  SaturateOnIntegerOverflow=on
  Abs1 : Abs  SaturateOnIntegerOverflow=on
  Abs3 : Abs  SaturateOnIntegerOverflow=on
  Add : Sum  Inputs=+-  SaturateOnIntegerOverflow=on  InputSameDT=on
  Add1 : Sum  Inputs=+-  SaturateOnIntegerOverflow=on  InputSameDT=on
  Add3 : Sum  Inputs=+-  SaturateOnIntegerOverflow=on  InputSameDT=on
  Constant1 : Constant  Value=AFS_facBstPresPT1_C
  Constant10 : Constant  Value=AFS_dnEngLdAdjThresHi_C
  Constant2 : Constant  Value=AFS_dpLdAdjThresHi_C
  Constant5 : Constant  Value=AFS_facQntCurrPT1_C
  Constant6 : Constant  Value=AFS_dqLdAdjThresHi_C
  Constant9 : Constant  Value=AFS_facnEngPT1_C
  Data Store Read1 : DataStoreRead  DataStoreName=AFS_VDDrftComp_DT
  Data Store Read2 : DataStoreRead  DataStoreName=AFS_VDDrftComp_DT
  Data Store Read4 : DataStoreRead  DataStoreName=AFS_VDDrftComp_DT
  Delay : Delay  DelayLength=1  InitialCondition=0
  Delay1 : Delay  DelayLength=1  InitialCondition=0
  Delay3 : Delay  DelayLength=1  InitialCondition=0
  Divide1 : Product  Inputs=*/  OutDataTypeStr=Inherit: Inherit via back propagation  SaturateOnIntegerOverflow=on
  Divide2 : Product  Inputs=*/  OutDataTypeStr=Inherit: Inherit via back propagation  SaturateOnIntegerOverflow=on
  Divide4 : Product  Inputs=*/  OutDataTypeStr=Inherit: Inherit via back propagation  SaturateOnIntegerOverflow=on
  PT1_S1 : CXLib/PT1_S16
  PT1_S16 : CXLib/PT1_S16
  PT1_S3 : CXLib/PT1_S16
  Relational Operator : RelationalOperator  Operator=<  OutDataTypeStr=boolean  RndMeth=Simplest  InputSameDT=on
  Relational Operator2 : RelationalOperator  Operator=<  OutDataTypeStr=boolean  RndMeth=Simplest  InputSameDT=on
  Relational Operator4 : RelationalOperator  Operator=<  OutDataTypeStr=boolean  RndMeth=Simplest  InputSameDT=on
  stBstPresGrad : Outport
  stGrad : Outport  Port=2
  stnEngGrad : Outport  Port=3
  wires:
  Relational Operator4/1 -> stnEngGrad/1
  Constant10/1 -> Relational Operator4/2
  PT1_S3/1 -> Relational Operator4/1  "AFS_dnEngAbsFlt_mp"
  Constant9/1 -> PT1_S3/1
  Abs3/1 -> PT1_S3/2  "AFS_dnEngAbs_mp"
  Divide4/1 -> Abs3/1
  Data Store Read4/1 -> Divide4/2
  Add3/1 -> Divide4/1
  Delay3/1 -> Add3/2
  Epm_nEng/1 -> Delay3/1, Add3/1
  Relational Operator2/1 -> stGrad/1
  Constant6/1 -> Relational Operator2/2
  PT1_S1/1 -> Relational Operator2/1  "AFS_dqCurrAbsFlt_mp"
  Constant5/1 -> PT1_S1/1
  Abs1/1 -> PT1_S1/2  "AFS_dqCurrAbs_mp"
  Divide2/1 -> Abs1/1
  Data Store Read2/1 -> Divide2/2
  Add1/1 -> Divide2/1
  Delay1/1 -> Add1/2
  InjCtl_qCurr/1 -> Delay1/1, Add1/1
  Relational Operator/1 -> stBstPresGrad/1
  Constant2/1 -> Relational Operator/2
  PT1_S16/1 -> Relational Operator/1  "AFS_dpIntValAbsFlt_mp"
  Constant1/1 -> PT1_S16/1
  Abs/1 -> PT1_S16/2  "AFS_dpIntValAbs_mp"
  Divide1/1 -> Abs/1
  Data Store Read1/1 -> Divide1/2
  Add/1 -> Divide1/1
  Delay/1 -> Add/2
  ASMod_pIndVol/1 -> Add/1, Delay/1

== system AFS_VDDrftComp/AFS_VDDrftComp/CalcCorFac/If Action Subsystem ==
  AFS_facCalcValFlt_mp : Inport
  AFS_dmAirMsFlt_mp : Inport  Port=2
  Action Port : ActionPort  ActionType=then
  Constant6 : Constant  Value=true  OutDataTypeStr=boolean
  Data Type Conversion : DataTypeConversion
  Data Type Conversion1 : DataTypeConversion
  Data Type Conversion2 : DataTypeConversion
  AFS_facCalcIdlAdjVal_mp : Outport
  AFS_dmIdlAirMs_mp : Outport  Port=2
  AFS_stCurrIdlAdj : Outport  Port=3
  wires:
  Data Type Conversion2/1 -> AFS_stCurrIdlAdj/1  "AFS_stCurrIdlAdj"
  Data Type Conversion1/1 -> AFS_dmIdlAirMs_mp/1  "AFS_dmIdlAirMs_mp"
  Data Type Conversion/1 -> AFS_facCalcIdlAdjVal_mp/1  "AFS_facCalcIdlAdjVal_mp"
  AFS_dmAirMsFlt_mp/1 -> Data Type Conversion1/1
  AFS_facCalcValFlt_mp/1 -> Data Type Conversion/1
  Constant6/1 -> Data Type Conversion2/1

== system AFS_VDDrftComp/AFS_VDDrftComp/CalcCorFac/If Action Subsystem1 ==
  AFS_facCalcValFlt_mp : Inport
  AFS_dmAirMsFlt_mp : Inport  Port=2
  Action Port : ActionPort  ActionType=then
  Constant6 : Constant  Value=true  OutDataTypeStr=boolean
  Data Type Conversion : DataTypeConversion
  Data Type Conversion1 : DataTypeConversion
  Data Type Conversion2 : DataTypeConversion
  AFS_facCalcLdAdjVal_mp : Outport
  AFS_dmLdAirMs_mp : Outport  Port=2
  AFS_stCurrLdAdj : Outport  Port=3
  wires:
  Data Type Conversion2/1 -> AFS_stCurrLdAdj/1  "AFS_stCurrLdAdj"
  Data Type Conversion1/1 -> AFS_dmLdAirMs_mp/1  "AFS_dmLdAirMs_mp"
  Data Type Conversion/1 -> AFS_facCalcLdAdjVal_mp/1  "AFS_facCalcLdAdjVal_mp"
  AFS_dmAirMsFlt_mp/1 -> Data Type Conversion1/1
  AFS_facCalcValFlt_mp/1 -> Data Type Conversion/1
  Constant6/1 -> Data Type Conversion2/1

== system AFS_VDDrftComp/AFS_VDDrftComp/UpdCorFac/Updata4 ==
  Action Port : ActionPort  ActionType=then
  Constant15 : Constant  Value=true  OutDataTypeStr=boolean
  stCurrAdj : Outport  InitialOutput=0
  wires:
  Constant15/1 -> stCurrAdj/1

== system AFS_VDDrftComp/AFS_VDDrftComp/UpdCorFac/update ==
  in : Inport
  Action Port : ActionPort  ActionType=then
  out : Outport
  wires:
  in/1 -> out/1  "AFS_facIdlAdjValUnLim_mp"

== system AFS_VDDrftComp/AFS_VDDrftComp/UpdCorFac/update1 ==
  in : Inport
  Action Port : ActionPort  ActionType=then
  out : Outport
  wires:
  in/1 -> out/1  "AFS_facLdAdjValUnLim_mp"

== system AFS_VDDrftComp/AFS_VDDrftComp/UpdCorFac/update2 ==
  in : Inport
  Action Port : ActionPort  ActionType=then
  out : Outport
  wires:
  in/1 -> out/1

== system AFS_VDDrftComp/AFS_VDDrftComp/UpdCorFac/update3 ==
  in : Inport
  Action Port : ActionPort  ActionType=then
  out : Outport
  wires:
  in/1 -> out/1
